simulink library "network"  (R2013b)
settings: Solver=ode45  StartTime=0.0  StopTime=10.0  RelTol=1e-3
values from neighbouring files (symbols this model uses):
  p_xmv = P+zeros(xmv_vec_length,1)    [Mode_1_Init.m]
undefined symbols (not defined in the file or in its folder): DMEAN, DVAR, IC, IC_x_star, p, randsrc
undefined symbols (not defined in the file): r_xmv, xmv_init
libraries: simulink x1
settings Model: Creator=rnc4  LastModifiedBy=rnc4

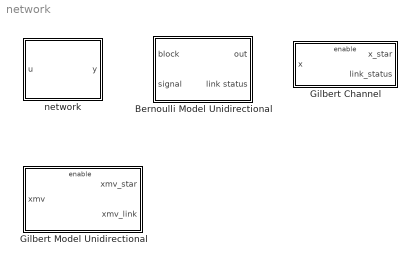
== system network ==
  Bernoulli Model Unidirectional : Subsystem  mask{P=0.1, X0=IC}
      mask prompts: P "Probability of Loss"; X0 "Initial condition:"
      mask TypeOptions X0: Memory/X0
      mask DialogControl DescTextVar Prompt: Set the probability P of packet loss.
  Gilbert Channel : Subsystem  TreatAsAtomicUnit=on  mask{IC_link_status=zeros(length(p),1), IC_x_star=IC_x_star, p=0.5, q=0.5}
      mask prompts: IC_link_status "Link status initial conditions:"; IC_x_star "Output initial conditions:"; p "Prob. remaining in good state:"; q "Prob. remaining in bad state:"
      mask TypeOptions IC_link_status: memory_link_status/X0
      mask TypeOptions IC_x_star: memory_x_star/X0
      mask TypeOptions p: const_p/Value
      mask TypeOptions q: const_r/Value
  Gilbert Model Unidirectional : Subsystem  AncestorBlock=network/Gilbert Model Bi-directional  mask{p=p_xmv, r=r_xmv, IC=xmv_init}
      mask prompts: p "Prob. of remaining in a good state:"; r "Prob. of remaining in a bad state:"; IC "Memory initial condition:"
      mask TypeOptions p: const_p_xmv/Value
      mask TypeOptions r: const_r_xmv/Value
      mask TypeOptions IC: xmv_memory/X0
  network : Subsystem  mask{WRITE_ENABLE=on, DMEAN=DMEAN, DVAR=DVAR, DMAX=10000, DMIN=0, Ns=1711, TSPACKET=0.01, InitialOutput=0, Filename=LOGFILE, MatrixName=net_log}
      mask prompts: WRITE_ENABLE "Enable logging"; DMEAN "Delay Mean"; DVAR "Delay Variance"; DMAX "Max Delay"; DMIN "Min Delay"; Ns "Random seed"; TSPACKET "Sample time"; InitialOutput "Initial output:"; Filename "File name:"; MatrixName "Variable name:"
      mask TypeOptions InitialOutput:
      | network
      | flight/InitialOutput
      mask TypeOptions Filename: Logger/Filename
      mask TypeOptions MatrixName: Logger/MatrixName
      mask DialogControl DescTextVar Prompt: This block provides network transport delay and logging capabillities.
      mask DialogControl cDelayParams Prompt: Delay
      mask DialogControl cLoggingParams Prompt: Logging
      mask Display:
      | image(imread('images/connect01.jpg'))
      | port_label('input',1,'u')
      | port_label('output',1,'y')

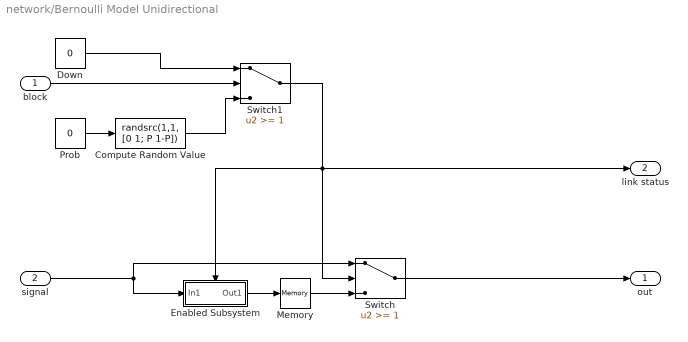
== system network/Bernoulli Model Unidirectional ==
  block : Inport
  signal : Inport  Port=2
  Compute Random Value : MATLABFcn  MATLABFcn=randsrc(1,1, [0 1; P 1-P])
  Down : Constant  Value=0
  Enabled Subsystem : Subsystem  TreatAsAtomicUnit=on
  Memory : Memory  X0=X0  InheritSampleTime=on
  Prob : Constant  Value=0
  Switch : Switch  Threshold=1
  Switch1 : Switch  Threshold=1
  out : Outport
  link status : Outport  Port=2
  wires:
  Switch1/1 -> Enabled Subsystem/Enable, Switch/2, link status/1
  Switch/1 -> out/1
  signal/1 -> Enabled Subsystem/1(In1), Switch/1
  Memory/1 -> Switch/3
  block/1 -> Switch1/2
  Compute Random Value/1 -> Switch1/3
  Down/1 -> Switch1/1
  Enabled Subsystem/1(Out1) -> Memory/1
  Prob/1 -> Compute Random Value/1

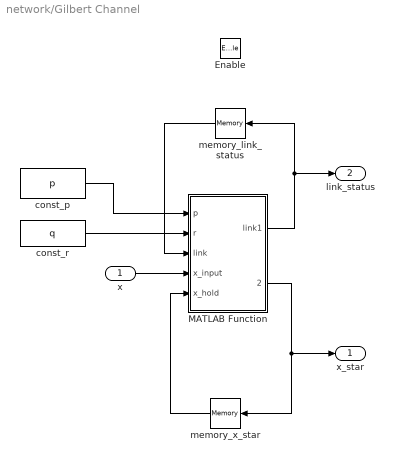
== system network/Gilbert Channel ==
  x : Inport
  Enable : EnablePort
  MATLAB Function : MATLAB Function  TreatAsAtomicUnit=on
  const_p : Constant  Value=p
  const_r : Constant  Value=q
  memory_link_status : Memory  X0=IC_link_status  InheritSampleTime=on  LinearizeAsDelay=on
  memory_x_star : Memory  X0=IC_x_star  InheritSampleTime=on  LinearizeAsDelay=on
  x_star : Outport
  link_status : Outport  Port=2
  wires:
  x/1 -> MATLAB Function/4(x_input)
  memory_x_star/1 -> MATLAB Function/5(x_hold)
  memory_link_status/1 -> MATLAB Function/3(link)
  MATLAB Function/2(x_output) -> x_star/1, memory_x_star/1
  MATLAB Function/1(link1) -> memory_link_status/1, link_status/1
  const_r/1 -> MATLAB Function/2(r)
  const_p/1 -> MATLAB Function/1(p)

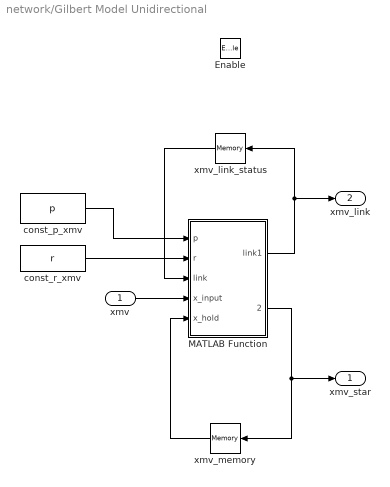
== system network/Gilbert Model Unidirectional ==
  xmv : Inport
  Enable : EnablePort
  MATLAB Function : MATLAB Function  TreatAsAtomicUnit=on
  const_p_xmv : Constant  Value=p
  const_r_xmv : Constant  Value=r
  xmv_link_status : Memory  X0=zeros(length(p_xmv),1)  InheritSampleTime=on  LinearizeAsDelay=on
  xmv_memory : Memory  X0=IC  InheritSampleTime=on  LinearizeAsDelay=on
  xmv_star : Outport
  xmv_link : Outport  Port=2
  wires:
  xmv/1 -> MATLAB Function/4(x_input)
  xmv_memory/1 -> MATLAB Function/5(x_hold)
  xmv_link_status/1 -> MATLAB Function/3(link)
  MATLAB Function/2(x_output) -> xmv_star/1, xmv_memory/1
  MATLAB Function/1(link1) -> xmv_link_status/1, xmv_link/1
  const_r_xmv/1 -> MATLAB Function/2(r)
  const_p_xmv/1 -> MATLAB Function/1(p)

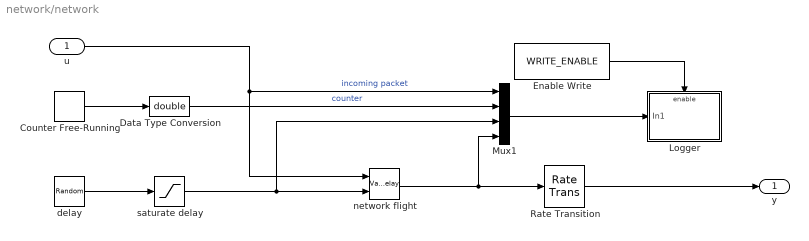
== system network/network ==
  u : Inport
  Counter Free-Running : simulink/Sources/Counter Free-Running  NumBits=32  tsamp=TSPACKET
  Data Type Conversion : DataTypeConversion  OutDataTypeStr=double
  Enable Write : Constant  Value=WRITE_ENABLE
  Logger : Subsystem  mask{MatrixName=net_log, Filename=LOGFILE}
      mask prompts: MatrixName "Variable name:"; Filename "File name:"
      mask TypeOptions MatrixName: To File/MatrixName
      mask TypeOptions Filename: To File/Filename
  Mux1 : Mux
  Rate Transition : RateTransition  OutPortSampleTime=TSPACKET
  delay : RandomNumber  Mean=DMEAN  Variance=DVAR  Seed=Ns  SampleTime=TSPACKET
      settings: AttributesFormatString=mean=%<Mean>\nvar=%<Variance>
  network flight : VariableTransportDelay  VariableDelayType=Variable transport delay  MaximumDelay=DMAX  InitialOutput=InitialOutput  MaximumPoints=2048
      settings: AttributesFormatString=|
      | Max Delay=%<MaximumDelay>
      | %<VariableDelayType>
  saturate delay : Saturate  UpperLimit=DMAX  LowerLimit=DMIN
      settings: AttributesFormatString=Dmax=%<UpperLimit>\nDlower=%<LowerLimit>
  y : Outport
  wires:
  u/1 -> network flight/1, Mux1/1  "incoming packet"
  Data Type Conversion/1 -> Mux1/2  "counter"
  Counter Free-Running/1 -> Data Type Conversion/1
  delay/1 -> saturate delay/1
  Mux1/1 -> Logger/1(In1)
  Enable Write/1 -> Logger/Enable
  Rate Transition/1 -> y/1
  network flight/1 -> Rate Transition/1, Mux1/4
  saturate delay/1 -> network flight/2, Mux1/3

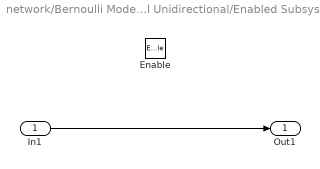
== system network/Bernoulli Model Unidirectional/Enabled Subsystem ==
  In1 : Inport
  Enable : EnablePort
  Out1 : Outport
  wires:
  In1/1 -> Out1/1

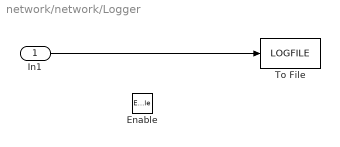
== system network/network/Logger ==
  In1 : Inport
  Enable : EnablePort
  To File : ToFile  Filename=LOGFILE  MatrixName=net_log
  wires:
  In1/1 -> To File/1

== matlab function network/Gilbert Channel/MATLAB Function ==
  data: p input; link1 output; r input; link input; x_output output; x_input input; x_hold input
function [link1,x_output] = fcn(p,r,link,x_input,x_hold)
x_output=link.*x_input+not(link).*x_hold;
link1=link;
for i=1:length(x_input);
    if link(i) == 1
        link1(i) = rand(1) > p(i);
    elseif link(i) == 0
        link1(i) = rand(1) > (1-r(i));
    end
end

== matlab function network/Gilbert Model Unidirectional/MATLAB Function ==
  data: p input; link1 output; r input; link input; x_output output; x_input input; x_hold input
function [link1,x_output] = fcn(p,r,link,x_input,x_hold)
x_output=link.*x_input+not(link).*x_hold;
link1=link;
for i=1:length(x_input);
    if link(i) == 1
    link1(i) = rand(1) > p(i);
    elseif link(i) == 0
    link1(i) = rand(1) > (1-r(i));
    end
end
